simulink model "ROS"  (R2018b)
settings: Solver=ode5  StartTime=0.0  StopTime=100  FixedStep=0.001  RelTol=1e-3  EnableMultiTasking=on
InitFcn:
  | clear
  | clear;
  | clc;
  | 
  | %create L1 and initial input x0
  | L1=[1 0 0 -1;-1 1 0 0;0 -1 1 0;0 0 -1 1];
  | I2=eye(2);
  | LK1=kron(L1,I2);
  | LK1=-LK1;
  | 
  | %E matrix
  | E=eye(8);
  | 
  | %axi of the sun
  | xd=[0 0 0 0 0 0 0 0];
  | 
  | %rounding speed
  | w0=1;
  | w_sun=0.05;
  | 
  | %init x0 and v0
  | x0=[1 3 2 1 3 2 4 5]';
  | v0=[1 1 2 1 1 1 1 1]';
  | xd=[20 20 30 20 30 10 20 10];
  | 
  | PID=[10,1,0,100];
StopFcn:
  | display('Result display:')
  | x1=x(:,2);
  | y1=x(:,3);
  | 
  | x2=x(:,4);
  | y2=x(:,5);
  | 
  | x3=x(:,6);
  | y3=x(:,7);
  | 
  | x4=x(:,8);
  | y4=x(:,9);
  | 
  | plot(x1,y1,x2,y2,x3,y3,x4,y4)
libraries: simulink x1
settings Model: Creator=richa  LastModifiedBy=108
settings OptimizationCC: LifeSpan=inf
settings DebuggingCC: SFUnexpectedBacktrackingDiag=warning  SFNoUnconditionalDefaultTransitionDiag=warning
settings SFSimCC: SimUseLocalCustomCode=off
settings RTWCC: RTWUseLocalCustomCode=off
settings CodeAppCC: StateflowObjectComments=on
settings GRTTargetCC: TargetLangStandard=C89/C90 (ANSI)  GeneratePreprocessorConditionals=Disable all
settings ConfigComp: CovMetricSettings=dw  CovHtmlReporting=on  CovSaveCumulativeToWorkspaceVar=on  CovSaveSingleToWorkspaceVar=on  CovExternalEMLEnable=off

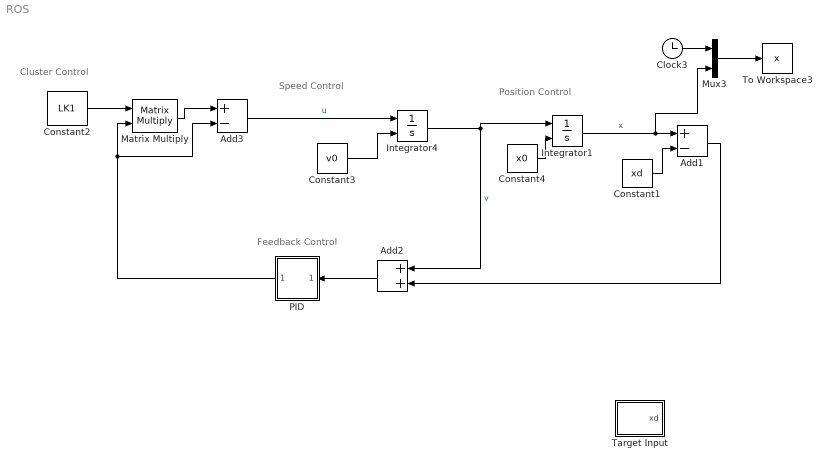
== system ROS ==
  note: Cluster Control
  note: Feedback Control
  note: Position Control
  note: Speed Control
  Add1 : Sum  Inputs=+-
  Add2 : Sum
  Add3 : Sum  Inputs=+-
  Clock3 : Clock
  Constant1 : Constant  Value=xd
  Constant2 : Constant  Value=LK1
  Constant3 : Constant  Value=v0
  Constant4 : Constant  Value=x0
  Integrator1 : Integrator  InitialConditionSource=external
  Integrator4 : Integrator  InitialConditionSource=external
  Matrix Multiply : Product  Multiplication=Matrix(*)
  Mux3 : Mux  Inputs=2
  PID : Subsystem
  Target Input : Subsystem
  To Workspace3 : ToWorkspace  VariableName=x  SampleTime=-1
  wires:
  Clock3/1 -> Mux3/1
  Add1/1 -> Add2/2
  Constant4/1 -> Integrator1/2
  Mux3/1 -> To Workspace3/1
  Constant3/1 -> Integrator4/2
  Integrator4/1 -> Integrator1/1, Add2/1  "v"
  Integrator1/1 -> Mux3/2, Add1/1  "x"
  Add2/1 -> PID/1(In1)
  PID/1(Out1) -> Matrix Multiply/2, Add3/2
  Add3/1 -> Integrator4/1  "u"
  Constant1/1 -> Add1/2
  Matrix Multiply/1 -> Add3/1
  Constant2/1 -> Matrix Multiply/1

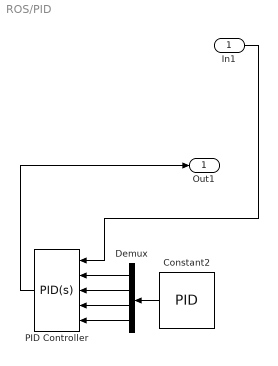
== system ROS/PID ==
  In1 : Inport
  Constant2 : Constant  Value=PID
  Demux : Demux
  PID Controller : simulink/Continuous/PID Controller  Controller=PID  Form=Parallel  TimeDomain=Continuous-time  SampleTime=-1  IntegratorMethod=Forward Euler  FilterMethod=Forward Euler  ControllerParametersSource=external  P=30  I=1  D=0  UseFilter=on  N=100  TunerSelectOption=Transfer Function Based (PID Tuner App)  InitialConditionSource=internal  InitialConditionForIntegrator=0  InitialConditionForFilter=0  DifferentiatorICPrevScaledInput=0  ExternalReset=none  TrackingMode=off  Kt=1  LimitOutput=off  UpperSaturationLimit=inf  LowerSaturationLimit=-inf  LinearizeAsGain=on  AntiWindupMode=none  Kb=1  POutMin=[]  POutMax=[]  IOutMin=[]  IOutMax=[]  DOutMin=[]  DOutMax=[]  NOutMin=[]  NOutMax=[]  SumOutMin=[]  SumOutMax=[]  SaturationOutMin=[]  SaturationOutMax=[]  PParamMin=[]  PParamMax=[]  IParamMin=[]  IParamMax=[]  DParamMin=[]  DParamMax=[]  NParamMin=[]  NParamMax=[]  KbParamMin=[]  KbParamMax=[]  KtParamMin=[]  KtParamMax=[]  KbOutMin=[]  KbOutMax=[]  KtOutMin=[]  KtOutMax=[]  IntegratorOutMin=[]  IntegratorOutMax=[]  FilterOutMin=[]  FilterOutMax=[]  SumI1OutMin=[]  SumI1OutMax=[]  SumI2OutMin=[]  SumI2OutMax=[]  SumI3OutMin=[]  SumI3OutMax=[]  SumI4OutMin=[]  SumI4OutMax=[]  SumDOutMin=[]  SumDOutMax=[]  DifferentiatorOutMin=[]  DifferentiatorOutMax=[]  FilterDiffOutCoefMin=[]  FilterDiffOutCoefMax=[]  ReciprocalOutMin=[]  ReciprocalOutMax=[]  SumDenOutMin=[]  SumDenOutMax=[]  SumNumOutMin=[]  SumNumOutMax=[]  DivideOutMin=[]  DivideOutMax=[]  IntegratorContinuousStateAttributes=''  IntegratorStateMustResolveToSignalObject=off  IntegratorRTWStateStorageClass=Auto  FilterContinuousStateAttributes=''  FilterStateMustResolveToSignalObject=off  FilterRTWStateStorageClass=Auto  ParallelPVariant=ExternalParameters  IdealPVariant=Disabled  IVariant=ExternalParameters  DVariant=ExternalParameters  IntegratorVariant=Continuous  SatVariant=Disabled  AWVariant=Passthrough  PCopyVariant=Disabled  TRVariant=Disabled  FdbkBlocksVariant=Forward  IdealPFdbkVariant=Disabled  SatFdbkVariant=Disabled  DerivativeFilterVariant=ContFilter  NVariant=ExternalParameters  NCopyVariant=Disabled  FilterICVariant=InternalICsFilter  IntegratorICVariant=InternalICs  ExternalResetVariant=Disabled  TRSumVariant=Passthrough  SumFdbkVariant=Disabled  SumVariant=Sum_PID
  Out1 : Outport
  wires:
  Demux/4 -> PID Controller/5
  Demux/3 -> PID Controller/4
  Demux/2 -> PID Controller/3
  Demux/1 -> PID Controller/2
  Constant2/1 -> Demux/1
  In1/1 -> PID Controller/1
  PID Controller/1 -> Out1/1

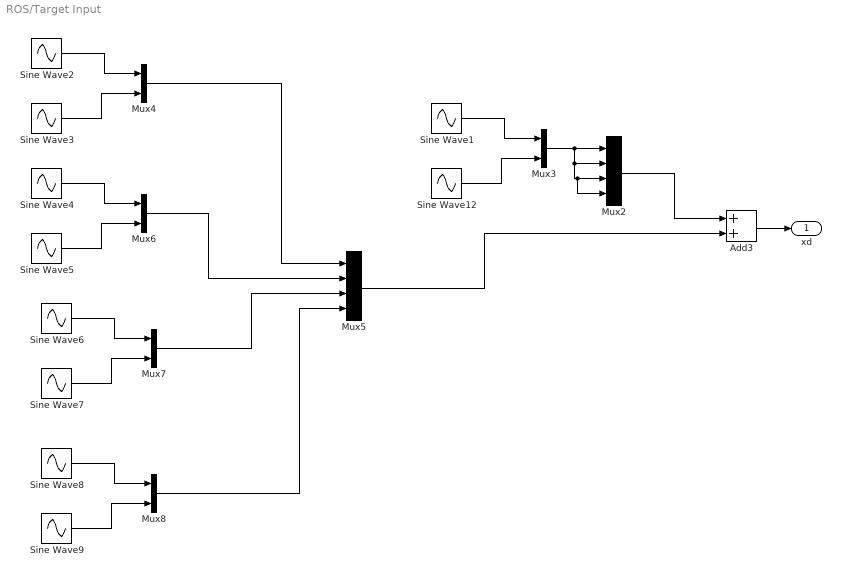
== system ROS/Target Input ==
  Add3 : Sum
  Mux2 : Mux
  Mux{3..4,6..8} (5 alike) : Mux  Inputs=2
  Mux5 : Mux
  Sine Wave1 : Sin  Amplitude=1000  Frequency=w_sun  SampleTime=0
  Sine Wave12 : Sin  Amplitude=1000  Frequency=w_sun  Phase=pi/2  SampleTime=0
  Sine Wave2 : Sin  Amplitude=100  Frequency=w0  SampleTime=0
  Sine Wave3 : Sin  Amplitude=100  Frequency=w0  Phase=pi/2  SampleTime=0
  Sine Wave4 : Sin  Amplitude=100  Frequency=w0  Phase=pi/2  SampleTime=0
  Sine Wave5 : Sin  Amplitude=100  Frequency=w0  Phase=pi  SampleTime=0
  Sine Wave6 : Sin  Amplitude=100  Frequency=w0  Phase=pi  SampleTime=0
  Sine Wave7 : Sin  Amplitude=100  Frequency=w0  Phase=pi*3/2  SampleTime=0
  Sine Wave8 : Sin  Amplitude=100  Frequency=w0  Phase=pi*3/2  SampleTime=0
  Sine Wave9 : Sin  Amplitude=100  Frequency=w0  Phase=2*pi  SampleTime=0
  xd : Outport
  wires:
  Add3/1 -> xd/1
  Sine Wave2/1 -> Mux4/1
  Sine Wave3/1 -> Mux4/2
  Mux4/1 -> Mux5/1
  Mux5/1 -> Add3/2
  Sine Wave4/1 -> Mux6/1
  Sine Wave5/1 -> Mux6/2
  Sine Wave6/1 -> Mux7/1
  Sine Wave7/1 -> Mux7/2
  Sine Wave8/1 -> Mux8/1
  Sine Wave9/1 -> Mux8/2
  Mux6/1 -> Mux5/2
  Mux7/1 -> Mux5/3
  Mux8/1 -> Mux5/4
  Mux2/1 -> Add3/1
  Sine Wave1/1 -> Mux3/1
  Sine Wave12/1 -> Mux3/2
  Mux3/1 -> Mux2/4, Mux2/3, Mux2/2, Mux2/1
